simulink model "MotorModel"  (R2019b)
settings: Solver=VariableStepAuto  StartTime=0.0  StopTime=10.0  RelTol=1e-3
undefined symbols (not defined in the file or in its folder): J_r, motor, sigbuilder_block, tau
libraries: cstblocks x1
settings Model: EnablePacing=on  Creator=miche  LastModifiedBy=miche

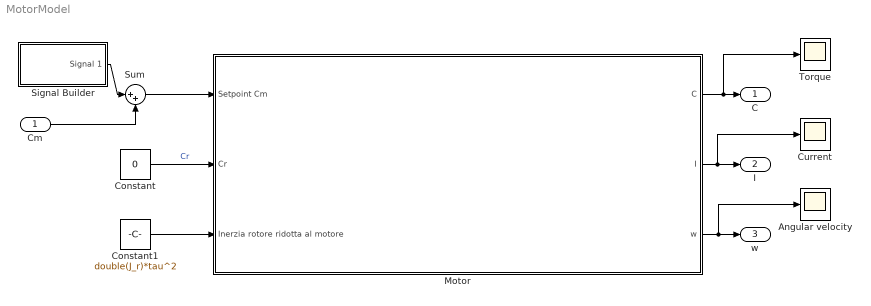
== system MotorModel ==
  Cm : Inport
  Angular velocity : Scope
  Constant : Constant  Value=0
  Constant1 : Constant  Value=double(J_r)*tau^2
  Current : Scope
  "Motor " : Subsystem
  Signal Builder : Subsystem  Tag=STV Subsys  LoadFcn=sigbuilder_block('load');  StartFcn=sigbuilder_block('start');  StopFcn=sigbuilder_block('stop');  ClipboardFcn=sigbuilder_block('clipboard');  mask(Sigbuilder block){tuvar=[0:10]}
      mask help: Simulink:masks:SigbuilderBlock_MD
      mask init:
      | if ~strcmp(get_param(bdroot(gcbh),'SimulationStatus'),'stopped') tuvar = sigbuilder_block('maskInit'); end
      settings: CopyFcn=sigbuilder_block('copy');  DeleteFcn=sigbuilder_block('delete');  ModelCloseFcn=sigbuilder_block('modelClose');  PreSaveFcn=sigbuilder_block('preSave');  PauseFcn=sigbuilder_block('pause');  ContinueFcn=sigbuilder_block('continue');  NameChangeFcn=sigbuilder_block('namechange');  OpenFcn=sigbuilder_block('open',[398.25 57.75 550.5 359.25 ]);  CloseFcn=sigbuilder_block('close');
      mask Display: plot(0, 0, 100, 100,[2, 2, 32, 32, 2], [68, 8, 8, 68, 68],[32, 2], [38, 38], [32, 19, 2],[53, 60, 44], [32, 17, 17, 2],[16, 16, 31, 31]);txt = getActiveGroup(gcbh);text(2, 100, txt,'verticalAlignment', 'top');
  Sum : Sum  Inputs=|++
  Torque : Scope
  C : Outport
  I : Outport  Port=2
  w : Outport  Port=3
  wires:
  Constant1/1 -> "Motor "/3(Inerzia rotore ridotta al motore)
  Constant/1 -> "Motor "/2(Cr)  "Cr"
  "Motor "/1("C ") -> Torque/1, C/1
  "Motor "/2("I ") -> Current/1, I/1
  "Motor "/3(w) -> Angular velocity/1, w/1
  Signal Builder/1(Signal 1) -> Sum/1
  Cm/1 -> Sum/2
  Sum/1 -> "Motor "/1(Setpoint Cm)

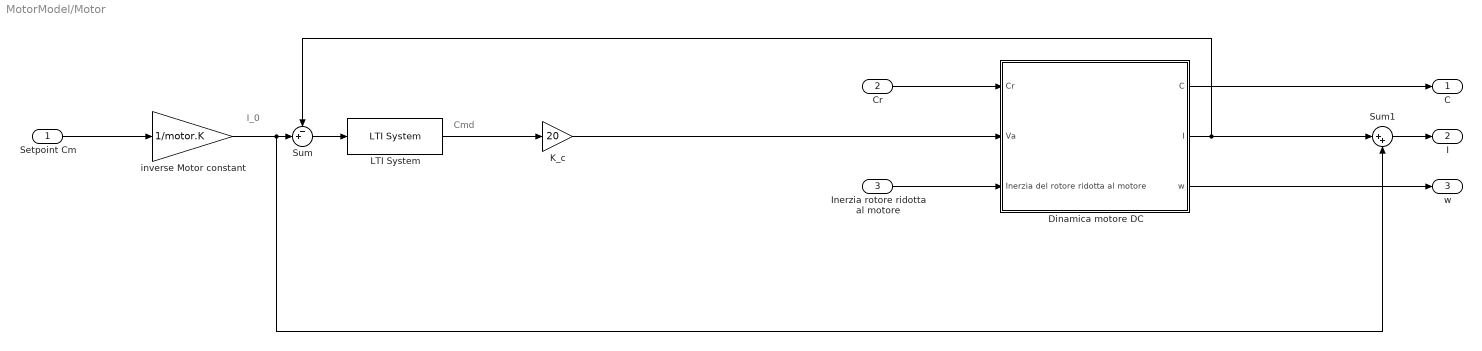
== system MotorModel/Motor  ==
  note: Cmd
  note: I_0
  Setpoint Cm : Inport
  Cr : Inport  Port=2
  Inerzia rotore ridotta al motore : Inport  Port=3
  Dinamica motore DC : Subsystem
  K_c : Gain  Gain=20
  LTI System : cstblocks/LTI System  sys=currentClosedLoop.PI_regulator  IC=[]
  Sum : Sum  Inputs=-+|
  Sum1 : Sum  Inputs=|++
  inverse Motor constant : Gain  Gain=1/motor.K
  "C " : Outport
  "I " : Outport  Port=2
  w : Outport  Port=3
  wires:
  inverse Motor constant/1 -> Sum1/2, Sum/2
  Setpoint Cm/1 -> inverse Motor constant/1
  Sum/1 -> LTI System/1
  LTI System/1 -> K_c/1
  Cr/1 -> Dinamica motore DC/1(Cr)
  K_c/1 -> Dinamica motore DC/2(Va)
  Inerzia rotore ridotta al motore/1 -> Dinamica motore DC/3(Inerzia del rotore ridotta al motore)
  Dinamica motore DC/1(C) -> "C "/1
  Dinamica motore DC/2(I) -> Sum1/1, Sum/1
  Sum1/1 -> "I "/1
  Dinamica motore DC/3(w) -> w/1

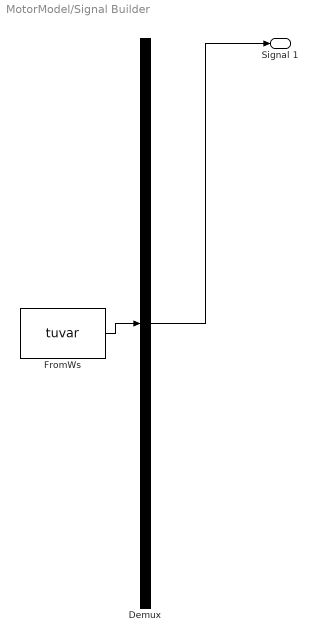
== system MotorModel/Signal Builder ==
  Demux : Demux  Tag=STV Demux  Outputs=1
  FromWs : FromWorkspace  Tag=STV FromWs  VariableName=tuvar  SampleTime=0
      SigBuilderData=|
      | common.afterFinalStr = 'Extrapolate'
      | common.sampleTime = 0
      | dataSet.timeRange = [0 10]
      | dataSet.name = 'Group 1'
      | sbobj.Groups.Name = 'Group 1'
      | sbobj.Groups.Signals.Name = 'Signal 1'
      | sbobj.Groups.Signals.XData = [0 0.01 0.01 0.1 0.1 10]
      | sbobj.Groups.Signals.YData = [28.1 28.1 29.1 29.1 28.1 28.1]
  Signal 1 : Outport  Tag=STV Outport
  wires:
  Demux/1 -> Signal 1/1
  FromWs/1 -> Demux/1

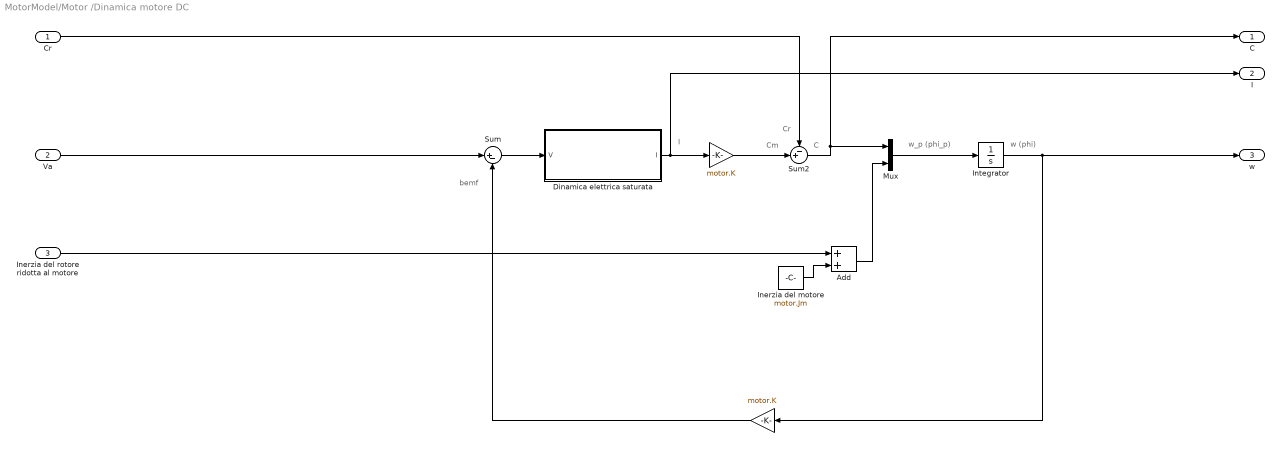
== system MotorModel/Motor /Dinamica motore DC ==
  note: w (phi)
  note: C
  note: I
  note: Cm
  note: Cr
  note: w_p (phi_p)
  note: bemf
  Cr : Inport
  Va : Inport  Port=2
  Inerzia del rotore ridotta al motore : Inport  Port=3
  " " : Gain  Gain=motor.K
  " " : Gain  Gain=motor.K
  Add : Sum
  "Dinamica elettrica saturata " : Subsystem
  Inerzia del motore : Constant  Value=motor.Jm
  Integrator : Integrator
  Mux : Mux  Inputs=2
  Sum : Sum  Inputs=|+-
  Sum2 : Sum  Inputs=-+|
  C : Outport
  I : Outport  Port=2
  w : Outport  Port=3
  wires:
  " "/1 -> Sum2/2
  Sum2/1 -> C/1, Mux/1
  Integrator/1 -> " "/1, w/1
  "Dinamica elettrica saturata "/1(I) -> I/1, " "/1
  Inerzia del motore/1 -> Add/2
  Inerzia del rotore ridotta al motore/1 -> Add/1
  Cr/1 -> Sum2/1
  " "/1 -> Sum/2
  Va/1 -> Sum/1
  Sum/1 -> "Dinamica elettrica saturata "/1(V)
  Mux/1 -> Integrator/1
  Add/1 -> Mux/2

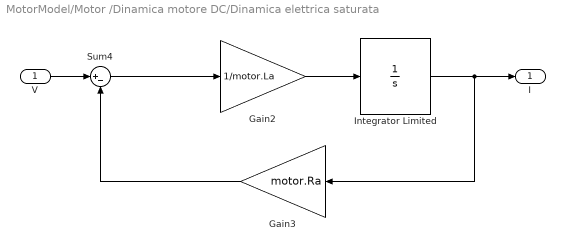
== system MotorModel/Motor /Dinamica motore DC/Dinamica elettrica saturata  ==
  V : Inport
  Gain2 : Gain  Gain=1/motor.La
  Gain3 : Gain  Gain=motor.Ra
  Integrator Limited : Integrator  LimitOutput=on  UpperSaturationLimit=motor.Imax  LowerSaturationLimit=-motor.Imax
  Sum4 : Sum  Inputs=|+-
  I : Outport
  wires:
  Gain3/1 -> Sum4/2
  Sum4/1 -> Gain2/1
  Gain2/1 -> Integrator Limited/1
  Integrator Limited/1 -> I/1, Gain3/1
  V/1 -> Sum4/1
